simulink model "test2"  (R2019b)
settings: Solver=VariableStepAuto  StartTime=0.0  StopTime=100  RelTol=1e-3
values from neighbouring files (symbols this model uses):
  fv1 = 1    [Untitled2.m]
  fv2 = 1    [Untitled2.m]
  fv3 = 1    [Untitled2.m]
  fv4 = 1    [Untitled2.m]
  K1 = 2000    [Ex_20.m]    (also in Ex_24.m = 0.5; Untitled2.m = 1)
  K2 = 25000    [Ex_20.m]    (also in Ex_24.m = 1; Untitled2.m = 1)
  M1 = 400    [Ex_20.m]    (also in Ex_21.m = 0.5; Untitled2.m = 1)
  M2 = 20    [Ex_20.m]    (also in Ex_21.m = 1; Untitled2.m = 1)
  M3 = 1    [Untitled2.m]
settings Model: Creator=andre  LastModifiedBy=Emanuel Pereira

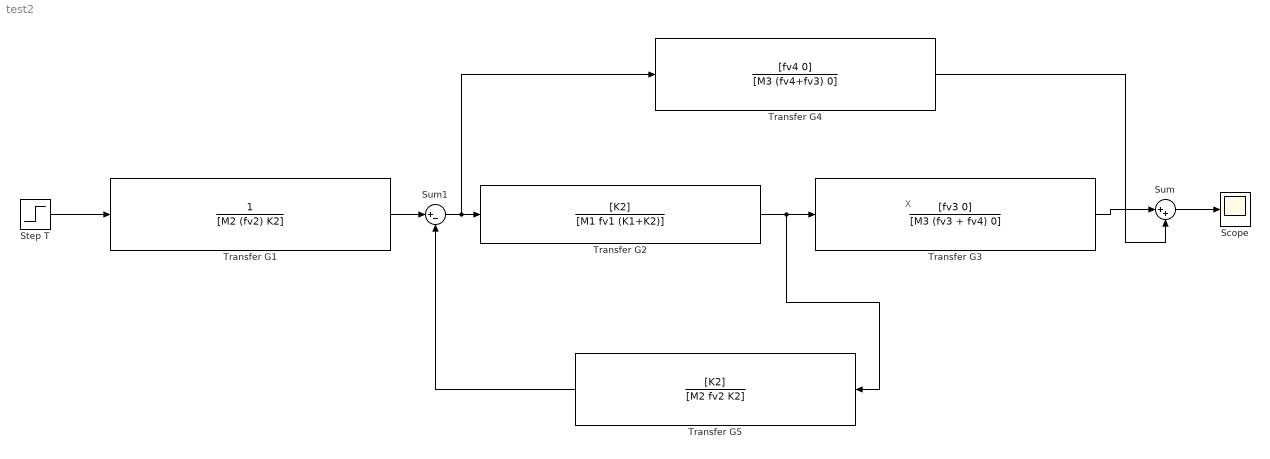
== system test2 ==
  note: X
  Scope : Scope
  Step T : Step  Time=0  SampleTime=0
  Sum : Sum  Inputs=|++
  Sum1 : Sum  Inputs=|+-
  Transfer G1 : TransferFcn  Denominator=[M2 (fv2) K2]
  Transfer G2 : TransferFcn  Numerator=[K2]  Denominator=[M1 fv1 (K1+K2)]
  Transfer G3 : TransferFcn  Numerator=[fv3 0]  Denominator=[M3 (fv3 + fv4) 0]
  Transfer G4 : TransferFcn  Numerator=[fv4 0]  Denominator=[M3 (fv4+fv3) 0]
  Transfer G5 : TransferFcn  Numerator=[K2]  Denominator=[M2 fv2 K2]
  wires:
  Sum/1 -> Scope/1
  Step T/1 -> Transfer G1/1
  Transfer G1/1 -> Sum1/1
  Sum1/1 -> Transfer G4/1, Transfer G2/1
  Transfer G2/1 -> Transfer G5/1, Transfer G3/1
  Transfer G4/1 -> Sum/2
  Transfer G3/1 -> Sum/1
  Transfer G5/1 -> Sum1/2
